simulink model "maxCalculatorTest"  (R2021b)
settings: Solver=FixedStepAuto  StartTime=0.0  StopTime=10.0  RelTol=1e-3
settings Model: Creator=lordx  LastModifiedBy=lordx
settings HardwareCC: TargetBitPerPointer=64  TargetBitPerSizeT=64  TargetBitPerPtrDiffT=64  TargetLongLongMode=on  TargetIntDivRoundTo=Zero  TargetEndianess=LittleEndian  TargetWordSize=64  TargetHWDeviceType=MATLAB Host  ProdEqTarget=off
settings RTWCC: Description=FMU based on RTW S-Function (Functional Mock-up Unit)  SystemTargetFile=rtwsfcnfmi.tlc  GenerateMakefile=off  TemplateMakefile=none  GenerateReport=on
settings CodeAppCC: ForceParamTrailComments=on  StateflowObjectComments=on  MATLABSourceComments=on
settings STFCustomTargetCC: TargetLangStandard=C99 (ISO)  ModelReferenceCompliant=off  CompOptLevelCompliant=on  MATLABClassNameForMDSCustomization=Simulink.SoftwareTarget.TargetSpecificTriggerConfigurationBase  SystemTargetFile=rtwsfcnfmi.tlc

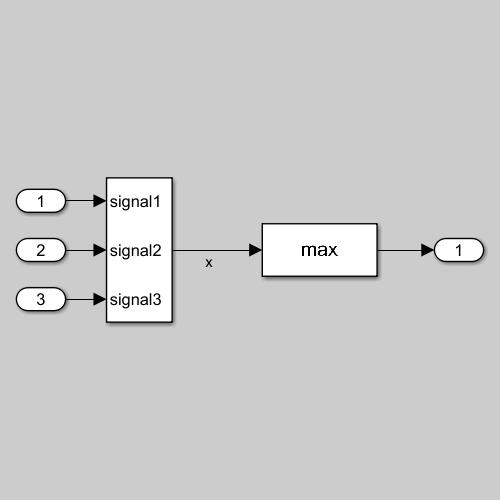
[thumbnail: Simulink's stored preview of the top-level diagram]
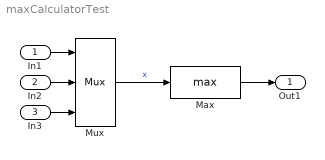
== system maxCalculatorTest ==
  In1 : Inport
  In2 : Inport  Port=2
  In3 : Inport  Port=3
  Max : MinMax  Function=max
  Mux : Mux  Inputs=3
      settings: DisplayOption=signals
  Out1 : Outport
  wires:
  In2/1 -> Mux/2
  In1/1 -> Mux/1
  In3/1 -> Mux/3
  Mux/1 -> Max/1  "x"
  Max/1 -> Out1/1
